simulink model "check_serial_close_loop_packet"  (R2020b)
settings: Solver=FixedStepDiscrete  StartTime=0.0  StopTime=inf  FixedStep=0.1  RelTol=1e-3
values from neighbouring files (symbols this model uses):
  tau = 1    [lpf_params.m]
  time_step = 0.1    [lpf_params.m]
undefined symbols (not defined in the file or in its folder): Serial_Port, Standard_Devices
libraries: sldrtlib x3
settings Model: Creator=Rahul Subramanian  LastModifiedBy=Rahul Subramanian

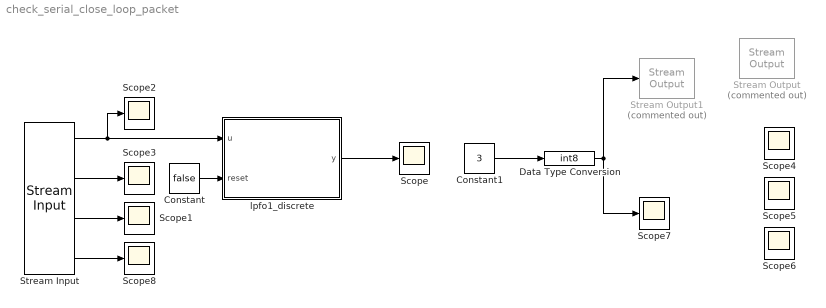
== system check_serial_close_loop_packet ==
  Constant : Constant  Value=false
  Constant1 : Constant  Value=3
  Data Type Conversion : DataTypeConversion  OutDataTypeStr=int8
  Scope{,1..8} (9 alike) : Scope
  Stream Input : sldrtlib/Stream Input  SampleTime=0.1  MaxMissedTicks=inf  ShowMissedTicks=on  YieldWhenWaiting=off  DrvName=Standard_Devices/Serial_Port  DrvAddress=4  DrvOptions=[19200 8 0 0 0 0 0 1]  DataTypes='int8'  FormatString='%d'  Terminator={'\n'}  ShowReady=on  ShowError=on
      settings: AttributesFormatString=Serial Port [4]  SourceProductBaseCode=WT
  Stream Output : sldrtlib/Stream Output  Commented=on  SampleTime=0.1  MaxMissedTicks=inf  ShowMissedTicks=on  YieldWhenWaiting=off  DrvName=Standard_Devices/Serial_Port  DrvAddress=4  DrvOptions=[9600 8 0 0 0 0 0 0]  PortSizes=1  FormatString='%d'  ShowReady=on  ShowError=on  InitialValue=[]  FinalValue=[]
      settings: AttributesFormatString=Serial Port [4]  SourceProductBaseCode=WT
  Stream Output1 : sldrtlib/Stream Output  Commented=on  SampleTime=0.1  MaxMissedTicks=10  ShowMissedTicks=off  YieldWhenWaiting=off  DrvName=Standard_Devices/Serial_Port  DrvAddress=4  DrvOptions=[9600 8 0 0 0 0 0 1]  PortSizes=[1]  FormatString='%d'  ShowReady=off  ShowError=off  InitialValue=[]  FinalValue='\n'
      settings: AttributesFormatString=Serial Port [4]  SourceProductBaseCode=WT
  lpfo1_discrete : Subsystem
  wires:
  Stream Input/1 -> Scope2/1, lpfo1_discrete/1(u)
  ? -> Scope4/1
  ? -> Scope5/1
  ? -> Scope6/1
  lpfo1_discrete/1(y) -> Scope/1
  Stream Input/2 -> Scope3/1
  Stream Input/3 -> Scope1/1
  Stream Input/4 -> Scope8/1
  Constant/1 -> lpfo1_discrete/2(reset)
  Data Type Conversion/1 -> Stream Output1/1, Scope7/1
  Constant1/1 -> Data Type Conversion/1

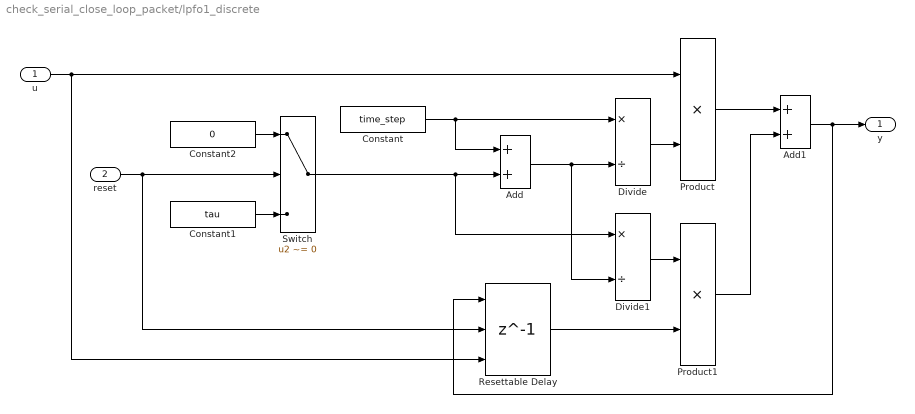
== system check_serial_close_loop_packet/lpfo1_discrete ==
  u : Inport
  reset : Inport  Port=2
  Add : Sum
  Add1 : Sum
  Constant : Constant  Value=time_step
  Constant1 : Constant  Value=tau
  Constant2 : Constant  Value=0
  Divide : Product  Inputs=*/
  Divide1 : Product  Inputs=*/
  Product : Product
  Product1 : Product
  Resettable Delay : Delay  DelayLength=1  InitialConditionSource=Input port  ExternalReset=Level
      settings: InputPortMap=u0,r5,p4
  Switch : Switch  Criteria=u2 ~= 0
  y : Outport
  wires:
  Constant/1 -> Add/1, Divide/1
  Divide/1 -> Product/2
  Switch/1 -> Divide1/1, Add/2
  Add1/1 -> y/1, Resettable Delay/1
  Add/1 -> Divide1/2, Divide/2
  u/1 -> Product/1, Resettable Delay/3
  Product/1 -> Add1/1
  Product1/1 -> Add1/2
  Divide1/1 -> Product1/1
  Constant2/1 -> Switch/1
  Constant1/1 -> Switch/3
  Resettable Delay/1 -> Product1/2
  reset/1 -> Switch/2, Resettable Delay/2
